simulink model "A1_p2_4_sim"  (R2019a)
settings: Solver=VariableStepAuto  StartTime=0.0  StopTime=100  RelTol=1e-3
undefined symbols (not defined in the file or in its folder): b, K, k_d, k_i, k_p, T, U, y_0
settings Model: Creator=paalthorseth  LastModifiedBy=paalthorseth

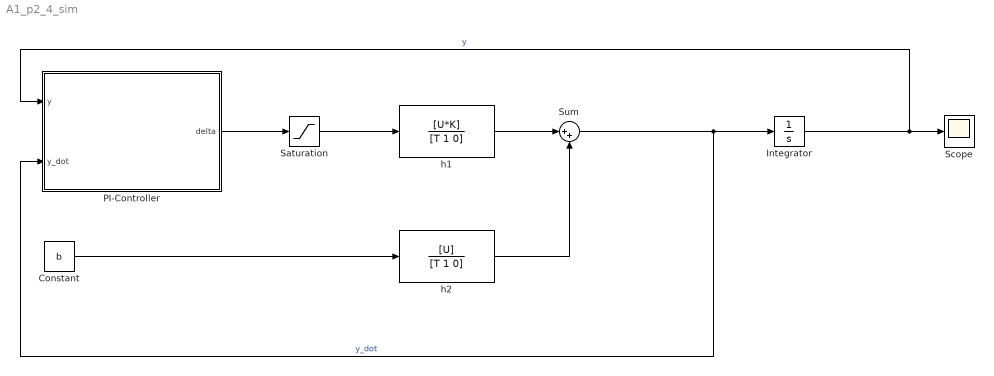
== system A1_p2_4_sim ==
  Constant : Constant  Value=b
  Integrator : Integrator  InitialCondition=y_0
  PI-Controller : Subsystem
  Saturation : Saturate  UpperLimit=20  LowerLimit=-20
  Scope : Scope
  Sum : Sum  Inputs=|++
  "h1 " : TransferFcn  Numerator=[U*K]  Denominator=[T 1 0]
  h2 : TransferFcn  Numerator=[U]  Denominator=[T 1 0]
  wires:
  PI-Controller/1(delta) -> Saturation/1
  Saturation/1 -> "h1 "/1
  Integrator/1 -> Scope/1, PI-Controller/1(y)  "y"
  "h1 "/1 -> Sum/1
  Sum/1 -> PI-Controller/2(y_dot), Integrator/1  "y_dot"
  Constant/1 -> h2/1
  h2/1 -> Sum/2

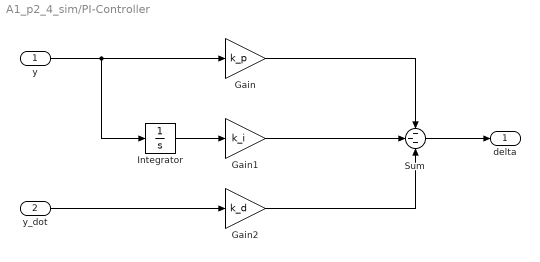
== system A1_p2_4_sim/PI-Controller ==
  y : Inport
  y_dot : Inport  Port=2
  Gain : Gain  Gain=k_p
  Gain1 : Gain  Gain=k_i
  Gain2 : Gain  Gain=k_d
  Integrator : Integrator
  Sum : Sum  Inputs=---
  delta : Outport
  wires:
  Sum/1 -> delta/1
  Integrator/1 -> Gain1/1
  Gain/1 -> Sum/1
  Gain1/1 -> Sum/2
  y/1 -> Integrator/1, Gain/1
  Gain2/1 -> Sum/3
  y_dot/1 -> Gain2/1
